simulink model "callback"  (Simulink 7.9)
settings: Solver=ode45  StartTime=0.0  StopTime=10.0  RelTol=1e-3
InitFcn:
  | t=(0:0.2:10)';
  | u=sin(t);
  | simin=[t u];
StopFcn:
  | figure,
  | plot(tout,yout);
settings Model: Creator=lenovo  LastModifiedBy=lenovo

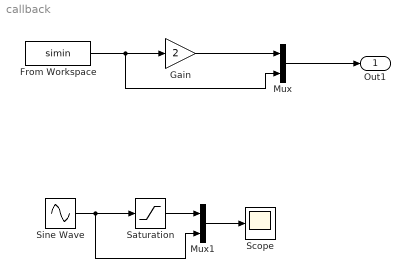
== system callback ==
  From Workspace : FromWorkspace  VariableName=simin  SampleTime=0
  Gain : Gain  Gain=2
  Mux : Mux  Inputs=2
  Mux1 : Mux  Inputs=2
  Saturation : Saturate
  Scope : Scope
  Sine Wave : Sin  StopFcn=|  SampleTime=0
      | blocks=find_system(bdroot,'BlockType','Scope');
      | for i=1:length(blocks)                         
      |    set_param(blocks{i},'Open','on');           
      | end
  Out1 : Outport
  wires:
  Gain/1 -> Mux/1
  From Workspace/1 -> Gain/1, Mux/2
  Mux/1 -> Out1/1
  Sine Wave/1 -> Saturation/1, Mux1/2
  Saturation/1 -> Mux1/1
  Mux1/1 -> Scope/1
